simulink model "Control_PD"  (R2018a)
settings: Solver=ode4  StartTime=0  StopTime=5000  FixedStep=ConfParam.confOrbit.dt  RelTol=1e-3
undefined symbols (not defined in the file): ConfParam, MTB
libraries: Estimator x2, CrossProd x2, ChangeFrame x2, Command x1, Date x1, KepOrbit x1, BdotController x1, OmegaError x1, Quat2Rot x1, Qerror x1, IGRF x1, SunEphemeris_MathWorks x1
settings Model: Creator=Cédric  LastModifiedBy=cedri
settings DataIOCC: SaveTime=off
settings DebuggingCC: MultiTaskRateTransMsg=warning

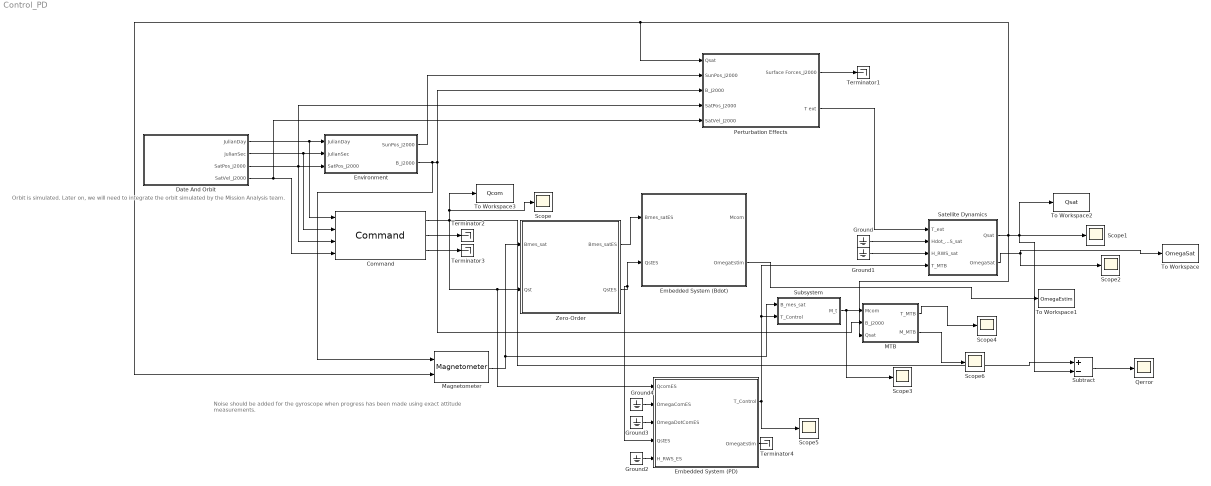
== system Control_PD ==
  note: Orbit is simulated. Later on, we will need to integrate the orbit simulated by the Mission Analysis team.
  note: Noise should be added for the gyroscope when progress has been made using exact attitude measurements.
  Command : Command/Command
  Date And Orbit : Subsystem
  Embedded System (Bdot) : Subsystem
  Embedded System (PD) : Subsystem
  Environment : Subsystem
  Ground{,1..4} (5 alike) : Ground
  MTB : Subsystem  AncestorBlock=MTB/MTB
  Magnetometer : Magnetometer/Magnetometer
  Perturbation Effects : Subsystem
  Qerror : Scope
  Satellite Dynamics : Subsystem  AncestorBlock=SatDyn/Satellite Dynamics
  Scope{,1..6} (7 alike) : Scope
  Subsystem : Subsystem
  Subtract : Sum  Inputs=+-
  Terminator{1..4} (4 alike) : Terminator
  To Workspace : ToWorkspace  VariableName=OmegaSat  SaveFormat=Timeseries  SampleTime=-1
  To Workspace1 : ToWorkspace  VariableName=OmegaEstim  SaveFormat=Timeseries  SampleTime=-1
  To Workspace2 : ToWorkspace  VariableName=Qsat  SaveFormat=Timeseries  SampleTime=-1
  To Workspace3 : ToWorkspace  VariableName=Qcom  SaveFormat=Timeseries  SampleTime=-1
  Zero-Order : Subsystem
  wires:
  Date And Orbit/1(JulianDay) -> Command/1, Environment/1(JulianDay)
  Date And Orbit/2(JulianSec) -> Command/2, Environment/2(JulianSec)
  Date And Orbit/3(SatPos_J2000) -> Perturbation Effects/4(SatPos_J2000), Command/3, Environment/3(SatPos_J2000)
  Environment/2(B_J2000) -> Magnetometer/1, MTB/2(B_J2000), Perturbation Effects/3(B_J2000)
  Date And Orbit/4(SatVel_J2000) -> Perturbation Effects/5(SatVel_J2000), Command/4
  Environment/1(SunPos_J2000) -> Perturbation Effects/2(SunPos_J2000)
  Zero-Order/1(Bmes_satES) -> Embedded System (Bdot)/1(Bmes_satES)
  Zero-Order/2(QstES) -> Embedded System (PD)/4(QstES), Embedded System (Bdot)/2(QstES)
  Perturbation Effects/2(T ext) -> Satellite Dynamics/1(T_ext)
  MTB/1(T_MTB) -> Scope4/1
  Magnetometer/1 -> Zero-Order/1(Bmes_sat), Subsystem/1(B_mes_sat)
  Command/1 -> Subtract/1, Scope/1, To Workspace3/1, Embedded System (PD)/1(QcomES), Zero-Order/2(Qst)
  Satellite Dynamics/1(Qsat) -> Subtract/2, Scope1/1, To Workspace2/1, Perturbation Effects/1(Qsat), Magnetometer/2, MTB/3(Qsat)
  Ground/1 -> Satellite Dynamics/2(Hdot_RWS_sat)
  Ground1/1 -> Satellite Dynamics/3(H_RWS_sat)
  MTB/2(M_MTB) -> Scope6/1
  Embedded System (Bdot)/2(OmegaEstim) -> To Workspace1/1
  Satellite Dynamics/2(OmegaSat) -> Scope2/1, To Workspace/1
  Perturbation Effects/1(Surface Forces_J2000) -> Terminator1/1
  Command/3 -> Terminator3/1
  Command/2 -> Terminator2/1
  Ground4/1 -> Embedded System (PD)/2(OmegaComES)
  Ground3/1 -> Embedded System (PD)/3(OmegaDotComES)
  Ground2/1 -> Embedded System (PD)/5(H_RWS_ES)
  Embedded System (PD)/2(OmegaEstim) -> Terminator4/1
  Embedded System (PD)/1(T_Control) -> Satellite Dynamics/4(T_MTB), Subsystem/2(T_Control), Scope5/1
  Subsystem/1(M_t) -> Scope3/1, MTB/1(Mcom)
  Subtract/1 -> Qerror/1

== system Control_PD/Date And Orbit ==
  Clock : Clock
  Current Simulation Date : Date/Current Simulation Date
  Orbit : KepOrbit/Keplerian Orbit
  JulianDay : Outport
  JulianSec : Outport  Port=2
  SatPos_J2000 : Outport  Port=3
  SatVel_J2000 : Outport  Port=4
  wires:
  Current Simulation Date/1 -> JulianDay/1
  Current Simulation Date/2 -> JulianSec/1
  Clock/1 -> Current Simulation Date/1
  Orbit/1 -> SatPos_J2000/1
  Orbit/2 -> SatVel_J2000/1

== system Control_PD/Embedded System (Bdot) ==
  Bmes_satES : Inport
  QstES : Inport  Port=2
  Estimator : Estimator/Estimator
  MTB controller : BdotController/Bdot Controller
  Mcom : Outport
  OmegaEstim : Outport  Port=2
  wires:
  QstES/1 -> Estimator/1
  Estimator/1 -> OmegaEstim/1
  Bmes_satES/1 -> MTB controller/1
  MTB controller/1 -> Mcom/1

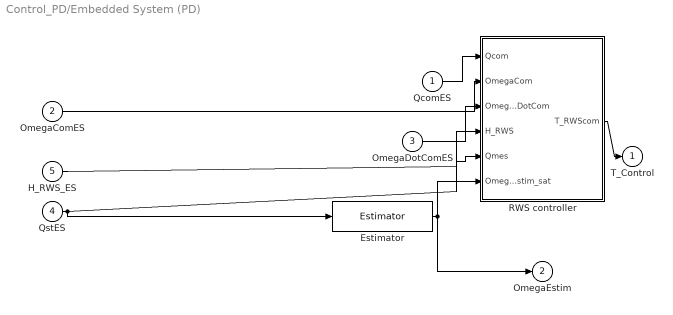
== system Control_PD/Embedded System (PD) ==
  QcomES : Inport
  OmegaComES : Inport  Port=2
  OmegaDotComES : Inport  Port=3
  QstES : Inport  Port=4
  H_RWS_ES : Inport  Port=5
  Estimator : Estimator/Estimator
  RWS controller : Subsystem  AncestorBlock=RWS_PDcontroller/RWS PD controller
  T_Control : Outport
  OmegaEstim : Outport  Port=2
  wires:
  QcomES/1 -> RWS controller/1(Qcom)
  OmegaDotComES/1 -> RWS controller/3(OmegaDotCom)
  RWS controller/1(T_RWScom) -> T_Control/1
  QstES/1 -> RWS controller/5(Qmes), Estimator/1
  H_RWS_ES/1 -> RWS controller/4(H_RWS)
  Estimator/1 -> RWS controller/6(OmegaEstim_sat), OmegaEstim/1
  OmegaComES/1 -> RWS controller/2(OmegaCom)

== system Control_PD/Environment ==
  JulianDay : Inport
  JulianSec : Inport  Port=2
  SatPos_J2000 : Inport  Port=3
  B J2000 : IGRF/IGRF in the J2000 frame
  Sun Ephemeris J2000 : SunEphemeris_MathWorks/Sun Ephemeris J2000
  SunPos_J2000 : Outport
  B_J2000 : Outport  Port=2
  wires:
  Sun Ephemeris J2000/1 -> SunPos_J2000/1
  JulianDay/1 -> Sun Ephemeris J2000/1, B J2000/1
  JulianSec/1 -> Sun Ephemeris J2000/2, B J2000/2
  SatPos_J2000/1 -> B J2000/3
  B J2000/1 -> B_J2000/1

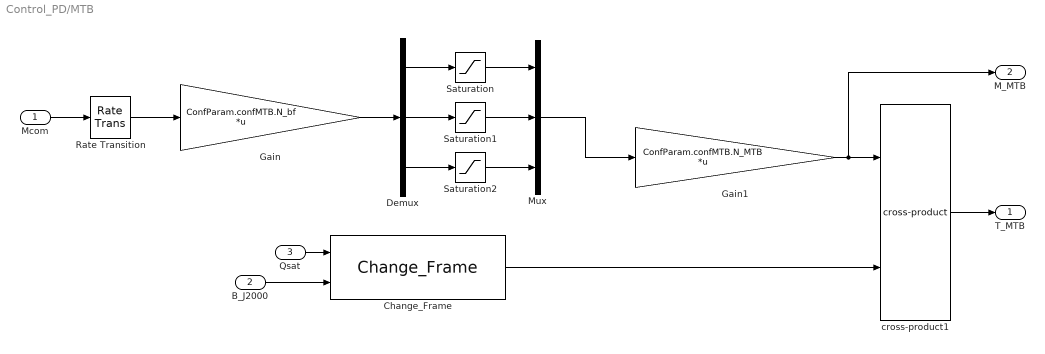
== system Control_PD/MTB ==
  Mcom : Inport
  B_J2000 : Inport  Port=2
  Qsat : Inport  Port=3
  Change_Frame : ChangeFrame/Change_Frame
  Demux : Demux  Outputs=3
  Gain : Gain  Gain=ConfParam.confMTB.N_bf  Multiplication=Matrix(K*u)
  Gain1 : Gain  Gain=ConfParam.confMTB.N_MTB  Multiplication=Matrix(K*u)
  Mux : Mux  Inputs=3
  Rate Transition : RateTransition  InitialCondition=[0;0;0]  OutPortSampleTime=ConfParam.confOrbit.dt
  Saturation : Saturate  UpperLimit=ConfParam.confMTB.M_max  LowerLimit=-ConfParam.confMTB.M_max
  Saturation1 : Saturate  UpperLimit=ConfParam.confMTB.M_max  LowerLimit=-ConfParam.confMTB.M_max
  Saturation2 : Saturate  UpperLimit=ConfParam.confMTB.M_max  LowerLimit=-ConfParam.confMTB.M_max
  cross-product1 : CrossProd/cross-product
  T_MTB : Outport
  M_MTB : Outport  Port=2
  wires:
  Change_Frame/1 -> cross-product1/2
  Qsat/1 -> Change_Frame/1
  Mcom/1 -> Rate Transition/1
  Gain1/1 -> M_MTB/1, cross-product1/1
  cross-product1/1 -> T_MTB/1
  B_J2000/1 -> Change_Frame/2
  Mux/1 -> Gain1/1
  Saturation2/1 -> Mux/3
  Saturation1/1 -> Mux/2
  Saturation/1 -> Mux/1
  Demux/2 -> Saturation1/1
  Demux/3 -> Saturation2/1
  Demux/1 -> Saturation/1
  Rate Transition/1 -> Gain/1
  Gain/1 -> Demux/1

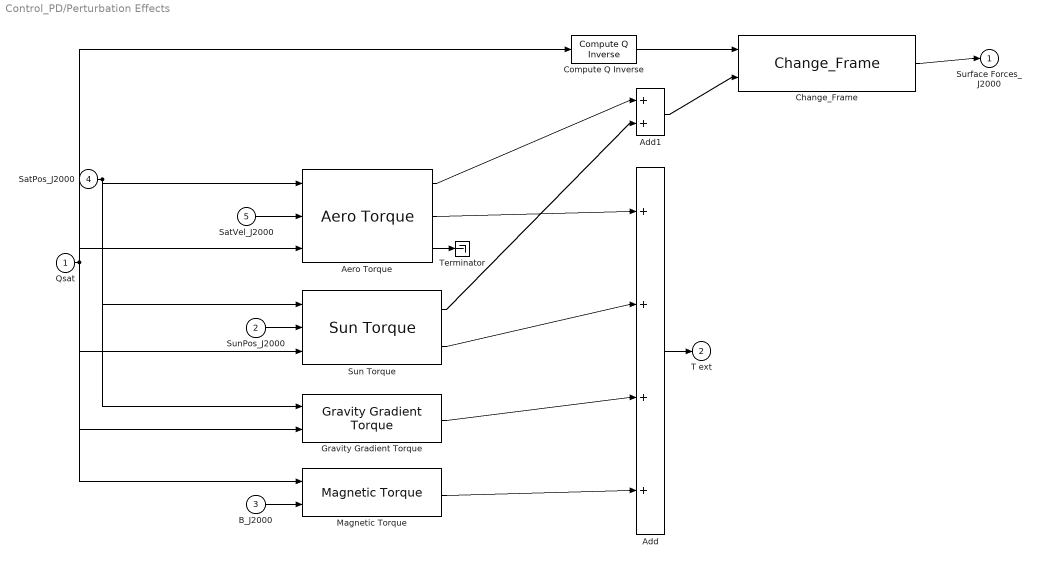
== system Control_PD/Perturbation Effects ==
  Qsat : Inport
  SunPos_J2000 : Inport  Port=2
  B_J2000 : Inport  Port=3
  SatPos_J2000 : Inport  Port=4
  SatVel_J2000 : Inport  Port=5
  Add : Sum  Inputs=++++
  Add1 : Sum
  Aero Torque : AeroTorqueA/Aero Torque
  Change_Frame : ChangeFrame/Change_Frame
  Compute Q Inverse : Qinverse/Compute Q Inverse
  Gravity Gradient Torque : GravGradTorque/Gravity Gradient Torque
  Magnetic Torque : MagnTorque/Magnetic Torque
  Sun Torque : SunTorqueA/Sun Torque
  Terminator : Terminator
  Surface Forces_J2000 : Outport
  T ext : Outport  Port=2
  wires:
  Compute Q Inverse/1 -> Change_Frame/1
  Change_Frame/1 -> Surface Forces_J2000/1
  Qsat/1 -> Compute Q Inverse/1, Gravity Gradient Torque/2, Sun Torque/3, Magnetic Torque/1, Aero Torque/3
  SunPos_J2000/1 -> Sun Torque/2
  B_J2000/1 -> Magnetic Torque/2
  SatPos_J2000/1 -> Sun Torque/1, Gravity Gradient Torque/1, Aero Torque/1
  SatVel_J2000/1 -> Aero Torque/2
  Aero Torque/3 -> Terminator/1
  Add1/1 -> Change_Frame/2
  Aero Torque/1 -> Add1/1
  Sun Torque/1 -> Add1/2
  Add/1 -> T ext/1
  Aero Torque/2 -> Add/1
  Sun Torque/2 -> Add/2
  Gravity Gradient Torque/1 -> Add/3
  Magnetic Torque/1 -> Add/4

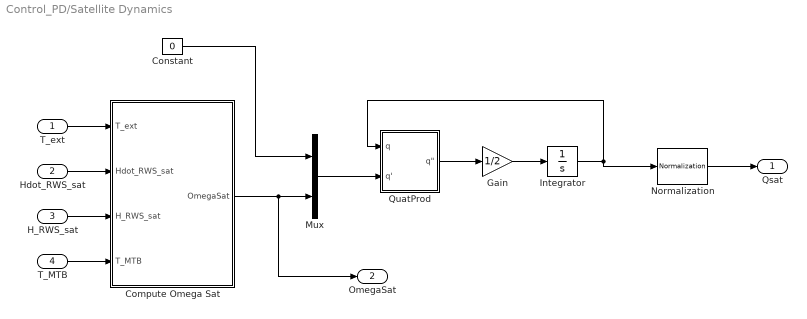
== system Control_PD/Satellite Dynamics ==
  T_ext : Inport
  Hdot_RWS_sat : Inport  Port=2
  H_RWS_sat : Inport  Port=3
  T_MTB : Inport  Port=4
  Compute Omega Sat : Subsystem
  Constant : Constant  Value=0
  Gain : Gain  Gain=1/2
  Integrator : Integrator  InitialCondition=ConfParam.confSatDyn.InitQsat
  Mux : Mux  Inputs=2
  Normalization : dspmathops/Normalization  NormType=Squared 2-norm  Bias=1e-10  NormOver=Each column  Dimension=1  roundingMode=Floor  overflowMode=off  accumDataTypeStr=Inherit: Same as product output  accumLastDataTypeStr=Inherit: Same as product output  outputDataTypeStr=Inherit: Same as product output  outputMin=[]  outputMax=[]  outputLastDataTypeStr=Inherit: Same as product output
      settings: SourceProductName=DSP System Toolbox
  QuatProd : Subsystem  TreatAsAtomicUnit=on
      settings: RTWFcnNameOpts=Use subsystem name  RTWFileNameOpts=Use subsystem name
  Qsat : Outport
  OmegaSat : Outport  Port=2
  wires:
  H_RWS_sat/1 -> Compute Omega Sat/3(H_RWS_sat)
  QuatProd/1("q\"") -> Gain/1
  T_MTB/1 -> Compute Omega Sat/4(T_MTB)
  Constant/1 -> Mux/1
  Hdot_RWS_sat/1 -> Compute Omega Sat/2(Hdot_RWS_sat)
  Gain/1 -> Integrator/1
  Integrator/1 -> QuatProd/1(q), Normalization/1
  Mux/1 -> QuatProd/2(q')
  Compute Omega Sat/1(OmegaSat) -> Mux/2, OmegaSat/1
  T_ext/1 -> Compute Omega Sat/1(T_ext)
  Normalization/1 -> Qsat/1

== system Control_PD/Subsystem ==
  B_mes_sat : Inport
  T_Control : Inport  Port=2
  MATLAB Function : MATLAB Function  TreatAsAtomicUnit=on
  M_t : Outport
  wires:
  B_mes_sat/1 -> MATLAB Function/1(B_vect)
  T_Control/1 -> MATLAB Function/2(T_c)
  MATLAB Function/1(M_t) -> M_t/1

== system Control_PD/Zero-Order ==
  Bmes_sat : Inport
  Qst : Inport  Port=2
  Zero-Order Hold : ZeroOrderHold  SampleTime=1/ConfParam.confES.frequency
  Zero-Order Hold1 : ZeroOrderHold  SampleTime=1/ConfParam.confES.frequency
  Bmes_satES : Outport
  QstES : Outport  Port=2
  wires:
  Bmes_sat/1 -> Zero-Order Hold/1
  Zero-Order Hold/1 -> Bmes_satES/1
  Qst/1 -> Zero-Order Hold1/1
  Zero-Order Hold1/1 -> QstES/1

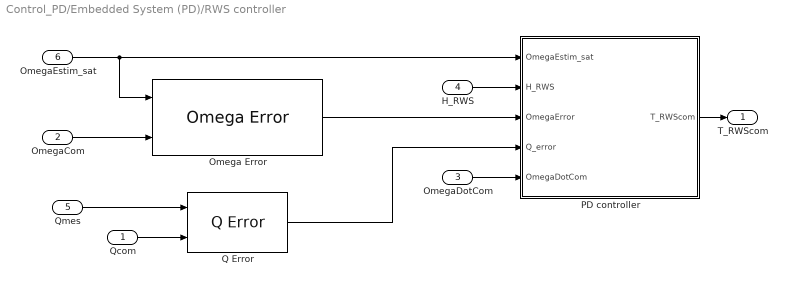
== system Control_PD/Embedded System (PD)/RWS controller ==
  Qcom : Inport
  OmegaCom : Inport  Port=2
  OmegaDotCom : Inport  Port=3
  H_RWS : Inport  Port=4
  Qmes : Inport  Port=5
  OmegaEstim_sat : Inport  Port=6
  Omega Error : OmegaError/Omega Error
  PD controller : Subsystem
  Q Error : Qerror/Q Error
  T_RWScom : Outport
  wires:
  OmegaCom/1 -> Omega Error/2
  OmegaEstim_sat/1 -> PD controller/1(OmegaEstim_sat), Omega Error/1
  Qmes/1 -> Q Error/1
  PD controller/1(T_RWScom) -> T_RWScom/1
  Omega Error/1 -> PD controller/3(OmegaError)
  H_RWS/1 -> PD controller/2(H_RWS)
  Qcom/1 -> Q Error/2
  Q Error/1 -> PD controller/4(Q_error)
  OmegaDotCom/1 -> PD controller/5(OmegaDotCom)

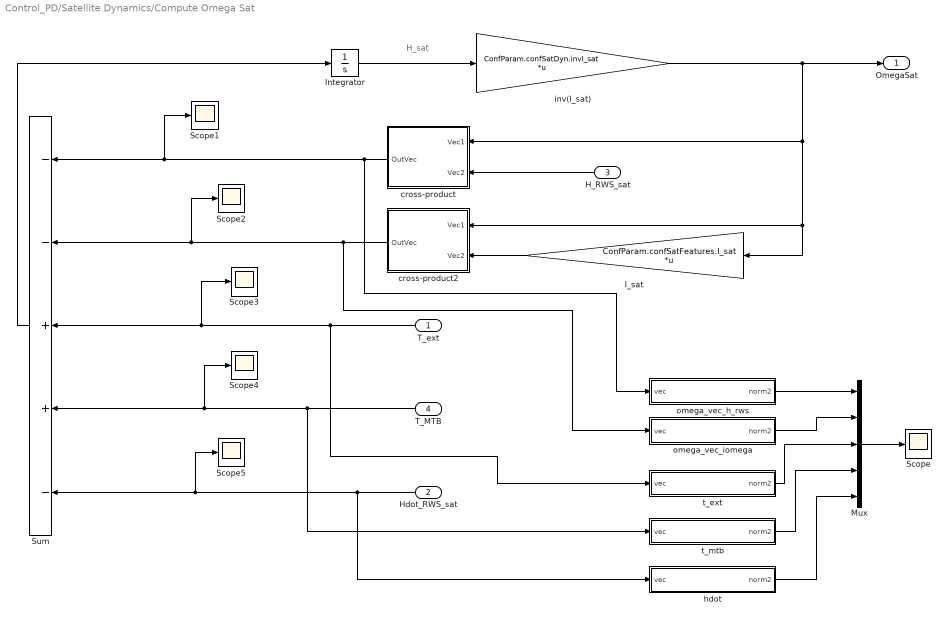
== system Control_PD/Satellite Dynamics/Compute Omega Sat ==
  note: H_sat
  T_ext : Inport
  Hdot_RWS_sat : Inport  Port=2
  H_RWS_sat : Inport  Port=3
  T_MTB : Inport  Port=4
  I_sat : Gain  Gain=ConfParam.confSatFeatures.I_sat  Multiplication=Matrix(K*u)
  Integrator : Integrator  InitialCondition=ConfParam.confSatFeatures.I_sat*ConfParam.confSatDyn.InitOmega_sat
  Mux : Mux  Inputs=5
  Scope{,1..5} (6 alike) : Scope
  Sum : Sum  Inputs=--++-
  cross-product : Subsystem
  cross-product2 : Subsystem
  hdot : Subsystem
  inv(I_sat) : Gain  Gain=ConfParam.confSatDyn.invI_sat  Multiplication=Matrix(K*u)
  omega_vec_h_rws : Subsystem
  omega_vec_iomega : Subsystem
  t_ext : Subsystem
  t_mtb : Subsystem
  OmegaSat : Outport
  wires:
  Mux/1 -> Scope/1
  H_RWS_sat/1 -> cross-product/2(Vec2)
  I_sat/1 -> cross-product2/2(Vec2)
  T_ext/1 -> t_ext/1(vec), Scope3/1, Sum/3
  T_MTB/1 -> t_mtb/1(vec), Sum/4, Scope4/1
  Sum/1 -> Integrator/1
  inv(I_sat)/1 -> OmegaSat/1, I_sat/1, cross-product2/1(Vec1), cross-product/1(Vec1)
  Integrator/1 -> inv(I_sat)/1
  hdot/1(norm2) -> Mux/5
  t_mtb/1(norm2) -> Mux/4
  t_ext/1(norm2) -> Mux/3
  omega_vec_iomega/1(norm2) -> Mux/2
  omega_vec_h_rws/1(norm2) -> Mux/1
  cross-product2/1(OutVec) -> Scope2/1, Sum/2, omega_vec_iomega/1(vec)
  cross-product/1(OutVec) -> Scope1/1, Sum/1, omega_vec_h_rws/1(vec)
  Hdot_RWS_sat/1 -> Scope5/1, Sum/5, hdot/1(vec)

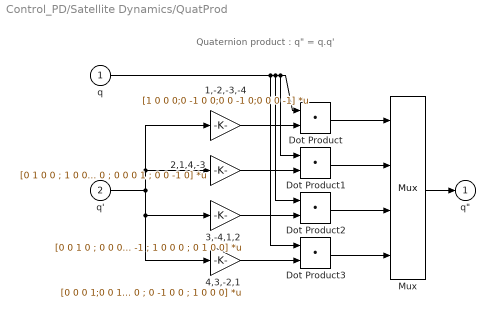
== system Control_PD/Satellite Dynamics/QuatProd ==
  note: Quaternion product : q" = q.q'
  q : Inport  OutDataTypeStr=double  PortDimensions=4
  q' : Inport  Port=2  OutDataTypeStr=double  PortDimensions=4
  1,-2,-3,-4 : Gain  Gain=[1 0 0 0;0 -1 0 0;0 0 -1 0;0 0 0 -1]  Multiplication=Matrix(K*u) (u vector)  SaturateOnIntegerOverflow=on  OutDataTypeStr=Inherit: Same as input  ParamDataTypeStr=Inherit: Same as input
  2,1,4,-3 : Gain  Gain=[0 1 0 0 ; 1 0 0 0 ; 0 0 0 1 ; 0 0 -1 0]  Multiplication=Matrix(K*u) (u vector)  SaturateOnIntegerOverflow=on  OutDataTypeStr=Inherit: Same as input  ParamDataTypeStr=Inherit: Same as input
  3,-4,1,2 : Gain  Gain=[0 0 1 0 ; 0 0 0 -1 ; 1 0 0 0 ; 0 1 0 0]  Multiplication=Matrix(K*u) (u vector)  SaturateOnIntegerOverflow=on  OutDataTypeStr=Inherit: Same as input  ParamDataTypeStr=Inherit: Same as input
  4,3,-2,1 : Gain  Gain=[0 0 0 1;0 0 1 0 ; 0 -1 0 0 ; 1 0 0 0]  Multiplication=Matrix(K*u) (u vector)  SaturateOnIntegerOverflow=on  OutDataTypeStr=Inherit: Same as input  ParamDataTypeStr=Inherit: Same as input
  Dot Product{,1..3} (4 alike) : DotProduct  InputSameDT=on  OutDataTypeStr=Inherit: Inherit via internal rule
  Mux : Mux
  "q\"" : Outport  OutDataTypeStr=double  PortDimensions=4  InitialOutput=0
  wires:
  Mux/1 -> "q\""/1
  Dot Product3/1 -> Mux/4
  Dot Product2/1 -> Mux/3
  Dot Product1/1 -> Mux/2
  Dot Product/1 -> Mux/1
  q/1 -> Dot Product3/1, Dot Product2/1, Dot Product1/1, Dot Product/1
  4,3,-2,1/1 -> Dot Product3/2
  3,-4,1,2/1 -> Dot Product2/2
  2,1,4,-3/1 -> Dot Product1/2
  1,-2,-3,-4/1 -> Dot Product/2
  q'/1 -> 2,1,4,-3/1, 1,-2,-3,-4/1, 4,3,-2,1/1, 3,-4,1,2/1

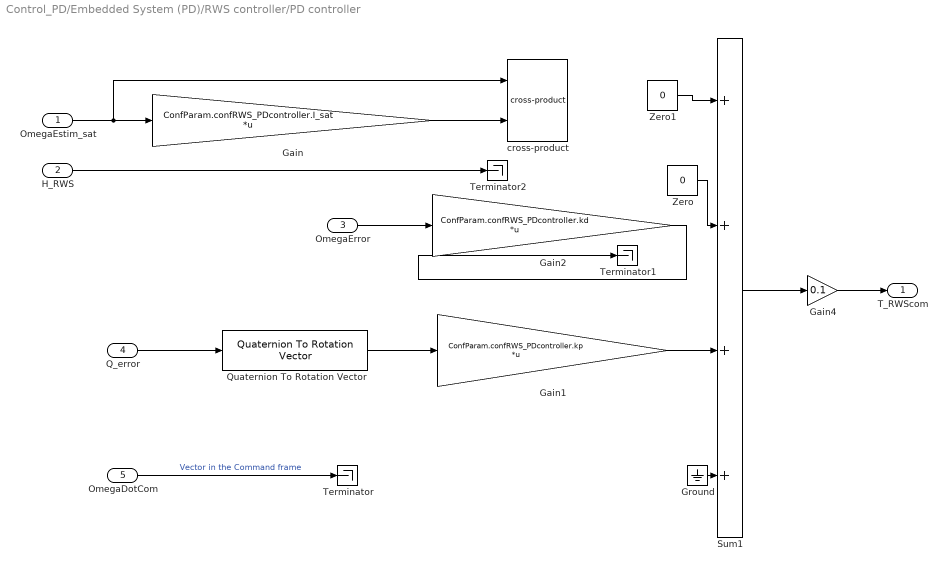
== system Control_PD/Embedded System (PD)/RWS controller/PD controller ==
  OmegaEstim_sat : Inport
  H_RWS : Inport  Port=2
  OmegaError : Inport  Port=3
  Q_error : Inport  Port=4
  OmegaDotCom : Inport  Port=5
  Gain : Gain  Gain=ConfParam.confRWS_PDcontroller.I_sat  Multiplication=Matrix(K*u)
  Gain1 : Gain  Gain=ConfParam.confRWS_PDcontroller.kp  Multiplication=Matrix(K*u)
  Gain2 : Gain  Gain=ConfParam.confRWS_PDcontroller.kd  Multiplication=Matrix(K*u)
  Gain4 : Gain  Gain=0.1
  Ground : Ground
  Quaternion To Rotation Vector : Quat2Rot/Quaternion To Rotation Vector
  Sum1 : Sum  Inputs=++++
  Terminator : Terminator
  Terminator1 : Terminator
  Terminator2 : Terminator
  Zero : Constant  Value=0
  Zero1 : Constant  Value=0
  cross-product : CrossProd/cross-product
  T_RWScom : Outport
  wires:
  Gain4/1 -> T_RWScom/1
  Sum1/1 -> Gain4/1
  OmegaDotCom/1 -> Terminator/1  "Vector in the Command frame"
  Gain1/1 -> Sum1/3
  Quaternion To Rotation Vector/1 -> Gain1/1
  H_RWS/1 -> Terminator2/1
  OmegaError/1 -> Gain2/1
  Q_error/1 -> Quaternion To Rotation Vector/1
  OmegaEstim_sat/1 -> Gain/1, cross-product/1
  Gain/1 -> cross-product/2
  Ground/1 -> Sum1/4
  Gain2/1 -> Terminator1/1
  Zero/1 -> Sum1/2
  Zero1/1 -> Sum1/1

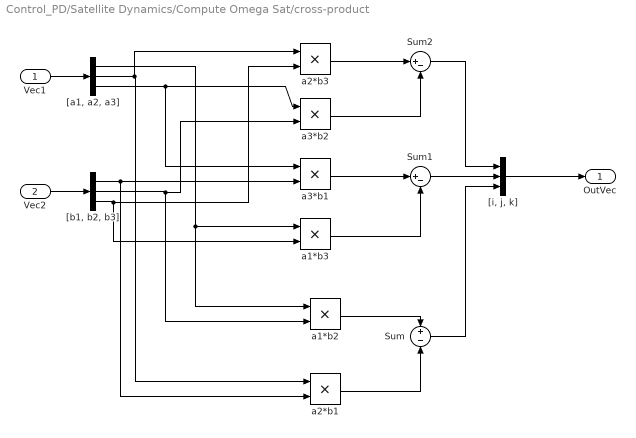
== system Control_PD/Satellite Dynamics/Compute Omega Sat/cross-product ==
  Vec1 : Inport
  Vec2 : Inport  Port=2
  Sum : Sum  Inputs=+-
  Sum1 : Sum  Inputs=|+-
  Sum2 : Sum  Inputs=|+-
  "[a1, a2, a3]" : Demux  Outputs=3
  "[b1, b2, b3]" : Demux  Outputs=3
  "[i, j, k]" : Mux  Inputs=3
  a1*b2 : Product
  a1*b3 : Product
  a2*b1 : Product
  a2*b3 : Product
  a3*b1 : Product
  a3*b2 : Product
  OutVec : Outport
  wires:
  Sum1/1 -> "[i, j, k]"/2
  Sum2/1 -> "[i, j, k]"/1
  Sum/1 -> "[i, j, k]"/3
  a3*b2/1 -> Sum2/2
  "[i, j, k]"/1 -> OutVec/1
  a1*b3/1 -> Sum1/2
  "[b1, b2, b3]"/3 -> a1*b3/2, a2*b3/2
  a2*b3/1 -> Sum2/1
  "[a1, a2, a3]"/3 -> a3*b2/1, a3*b1/1
  a3*b1/1 -> Sum1/1
  a1*b2/1 -> Sum/1
  "[b1, b2, b3]"/2 -> a1*b2/2, a3*b2/2
  Vec1/1 -> "[a1, a2, a3]"/1
  "[a1, a2, a3]"/1 -> a1*b2/1, a1*b3/1
  Vec2/1 -> "[b1, b2, b3]"/1
  "[a1, a2, a3]"/2 -> a2*b1/1, a2*b3/1
  "[b1, b2, b3]"/1 -> a2*b1/2, a3*b1/2
  a2*b1/1 -> Sum/2

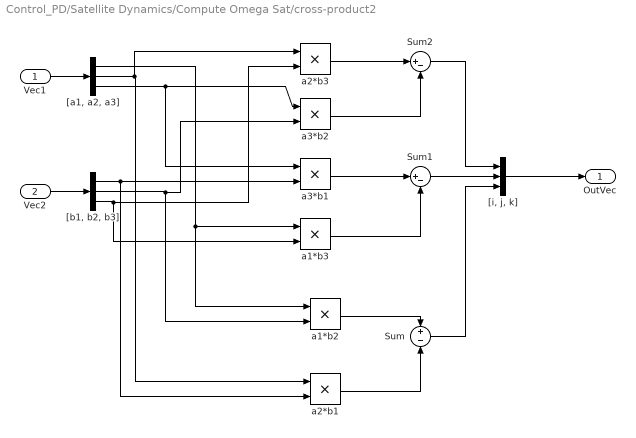
== system Control_PD/Satellite Dynamics/Compute Omega Sat/cross-product2 ==
  Vec1 : Inport
  Vec2 : Inport  Port=2
  Sum : Sum  Inputs=+-
  Sum1 : Sum  Inputs=|+-
  Sum2 : Sum  Inputs=|+-
  "[a1, a2, a3]" : Demux  Outputs=3
  "[b1, b2, b3]" : Demux  Outputs=3
  "[i, j, k]" : Mux  Inputs=3
  a1*b2 : Product
  a1*b3 : Product
  a2*b1 : Product
  a2*b3 : Product
  a3*b1 : Product
  a3*b2 : Product
  OutVec : Outport
  wires:
  Sum1/1 -> "[i, j, k]"/2
  Sum2/1 -> "[i, j, k]"/1
  Sum/1 -> "[i, j, k]"/3
  a3*b2/1 -> Sum2/2
  "[i, j, k]"/1 -> OutVec/1
  a1*b3/1 -> Sum1/2
  "[b1, b2, b3]"/3 -> a1*b3/2, a2*b3/2
  a2*b3/1 -> Sum2/1
  "[a1, a2, a3]"/3 -> a3*b2/1, a3*b1/1
  a3*b1/1 -> Sum1/1
  a1*b2/1 -> Sum/1
  "[b1, b2, b3]"/2 -> a1*b2/2, a3*b2/2
  Vec1/1 -> "[a1, a2, a3]"/1
  "[a1, a2, a3]"/1 -> a1*b2/1, a1*b3/1
  Vec2/1 -> "[b1, b2, b3]"/1
  "[a1, a2, a3]"/2 -> a2*b1/1, a2*b3/1
  "[b1, b2, b3]"/1 -> a2*b1/2, a3*b1/2
  a2*b1/1 -> Sum/2

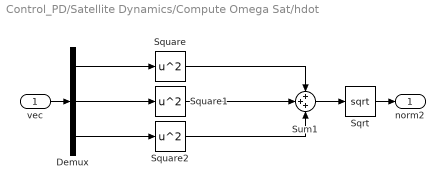
== system Control_PD/Satellite Dynamics/Compute Omega Sat/hdot ==
  vec : Inport
  Demux : Demux  Outputs=3
  Sqrt : Sqrt  SaturateOnIntegerOverflow=on
  Square : Math  Operator=square  SaturateOnIntegerOverflow=on
  Square1 : Math  Operator=square  SaturateOnIntegerOverflow=on
  Square2 : Math  Operator=square  SaturateOnIntegerOverflow=on
  Sum1 : Sum  Inputs=3
  norm2 : Outport
  wires:
  vec/1 -> Demux/1
  Sqrt/1 -> norm2/1
  Demux/2 -> Square1/1
  Square/1 -> Sum1/1
  Demux/3 -> Square2/1
  Square2/1 -> Sum1/3
  Square1/1 -> Sum1/2
  Demux/1 -> Square/1
  Sum1/1 -> Sqrt/1

== system Control_PD/Satellite Dynamics/Compute Omega Sat/omega_vec_h_rws ==
  vec : Inport
  Demux : Demux  Outputs=3
  Sqrt : Sqrt  SaturateOnIntegerOverflow=on
  Square : Math  Operator=square  SaturateOnIntegerOverflow=on
  Square1 : Math  Operator=square  SaturateOnIntegerOverflow=on
  Square2 : Math  Operator=square  SaturateOnIntegerOverflow=on
  Sum1 : Sum  Inputs=3
  norm2 : Outport
  wires:
  vec/1 -> Demux/1
  Sqrt/1 -> norm2/1
  Demux/2 -> Square1/1
  Square/1 -> Sum1/1
  Demux/3 -> Square2/1
  Square2/1 -> Sum1/3
  Square1/1 -> Sum1/2
  Demux/1 -> Square/1
  Sum1/1 -> Sqrt/1

== system Control_PD/Satellite Dynamics/Compute Omega Sat/omega_vec_iomega ==
  vec : Inport
  Demux : Demux  Outputs=3
  Sqrt : Sqrt  SaturateOnIntegerOverflow=on
  Square : Math  Operator=square  SaturateOnIntegerOverflow=on
  Square1 : Math  Operator=square  SaturateOnIntegerOverflow=on
  Square2 : Math  Operator=square  SaturateOnIntegerOverflow=on
  Sum1 : Sum  Inputs=3
  norm2 : Outport
  wires:
  vec/1 -> Demux/1
  Sqrt/1 -> norm2/1
  Demux/2 -> Square1/1
  Square/1 -> Sum1/1
  Demux/3 -> Square2/1
  Square2/1 -> Sum1/3
  Square1/1 -> Sum1/2
  Demux/1 -> Square/1
  Sum1/1 -> Sqrt/1

== system Control_PD/Satellite Dynamics/Compute Omega Sat/t_ext ==
  vec : Inport
  Demux : Demux  Outputs=3
  Sqrt : Sqrt  SaturateOnIntegerOverflow=on
  Square : Math  Operator=square  SaturateOnIntegerOverflow=on
  Square1 : Math  Operator=square  SaturateOnIntegerOverflow=on
  Square2 : Math  Operator=square  SaturateOnIntegerOverflow=on
  Sum1 : Sum  Inputs=3
  norm2 : Outport
  wires:
  vec/1 -> Demux/1
  Sqrt/1 -> norm2/1
  Demux/2 -> Square1/1
  Square/1 -> Sum1/1
  Demux/3 -> Square2/1
  Square2/1 -> Sum1/3
  Square1/1 -> Sum1/2
  Demux/1 -> Square/1
  Sum1/1 -> Sqrt/1

== system Control_PD/Satellite Dynamics/Compute Omega Sat/t_mtb ==
  vec : Inport
  Demux : Demux  Outputs=3
  Sqrt : Sqrt  SaturateOnIntegerOverflow=on
  Square : Math  Operator=square  SaturateOnIntegerOverflow=on
  Square1 : Math  Operator=square  SaturateOnIntegerOverflow=on
  Square2 : Math  Operator=square  SaturateOnIntegerOverflow=on
  Sum1 : Sum  Inputs=3
  norm2 : Outport
  wires:
  vec/1 -> Demux/1
  Sqrt/1 -> norm2/1
  Demux/2 -> Square1/1
  Square/1 -> Sum1/1
  Demux/3 -> Square2/1
  Square2/1 -> Sum1/3
  Square1/1 -> Sum1/2
  Demux/1 -> Square/1
  Sum1/1 -> Sqrt/1

== matlab function Control_PD/Subsystem/MATLAB Function ==
  data: B_vect input; M_t output; T_c input
% Computing of the magnetic moment to apply to the magnetorquer,
% given the control torque
function M_t = fcn(B_vect, T_c)
    B_mat = [0, B_vect(3), -B_vect(2);
            - B_vect(3), 0, B_vect(1);
            B_vect(2), -B_vect(1), 0];
    % Correction factor for B singualarity
%     m = sqrt(det(B_mat' * B_mat));
%     m0 = 1e-5;
%     lam0 = 1 ;
%     if m > m0
%         k = lam0 * (1 - m/m0)^2;
%     else
%         k = 0;  
%     end
    k = 1e-7;
        
    % Matricial form of the B vector for the crossproduct
    
    
    
    M_t = (B_mat'*B_mat + k * eye(3)) \ B_mat' * T_c;
end
